simulink model "Flexible_State_Space_Sim"  (R2021a)
settings: Solver=VariableStepAuto  StartTime=0.0  StopTime=2.5  RelTol=1e-3
settings Model: Creator=USER  LastModifiedBy=USER

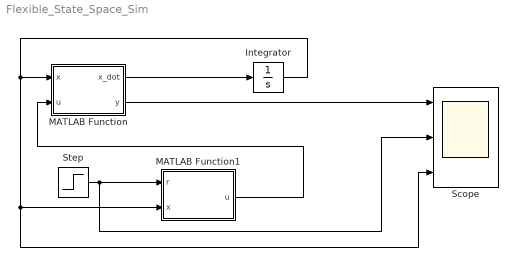
== system Flexible_State_Space_Sim ==
  Integrator : Integrator  InitialCondition=zeros(4,1)
  MATLAB Function : MATLAB Function  TreatAsAtomicUnit=on
  MATLAB Function1 : MATLAB Function  TreatAsAtomicUnit=on
  Scope : Scope  NumInputPorts=3
  Step : Step  Time=0  SampleTime=0
  wires:
  MATLAB Function/1(x_dot) -> Integrator/1
  Integrator/1 -> Scope/3, MATLAB Function1/2(x), MATLAB Function/1(x)
  Step/1 -> Scope/2, MATLAB Function1/1(r)
  MATLAB Function1/1(u) -> MATLAB Function/2(u)
  MATLAB Function/2(y) -> Scope/1

== matlab function Flexible_State_Space_Sim/MATLAB Function ==
  data: x input; x_dot output; u input; y output
function [x_dot, y]= fcn(x, u)

A = [0, 0, 1,0; 0, 0, 0, 1; 0, 483.13, -28.26, 0; 0, -837.21, 28.26, 0];
B = [0; 0; 49.7; -49.7];
C = [1, 0, 0, 0; 0, 1, 0, 0];
D = [0; 0];
x_dot = A*x + B*u;
y = C*x + D*u;

end

== matlab function Flexible_State_Space_Sim/MATLAB Function1 ==
  data: r input; u output; x input
function u = fcn(r, x)

k = [14.726713477884898,-1.004970587756365e+02,2.737188003188594,0.084874119888797];
u = r - k*x;

end
